simulink model "motor_position_pid_controller"  (R2020a)
settings: Solver=VariableStepAuto  StartTime=0.0  StopTime=10.0  RelTol=1e-3
undefined symbols (not defined in the file or in its folder): B, J, K, L, R
settings Model: DataDictionary=data_dict_motorposition.sldd  Creator=kiran  LastModifiedBy=kiran
settings DataIOCC: SaveOutput=off  SaveTime=off

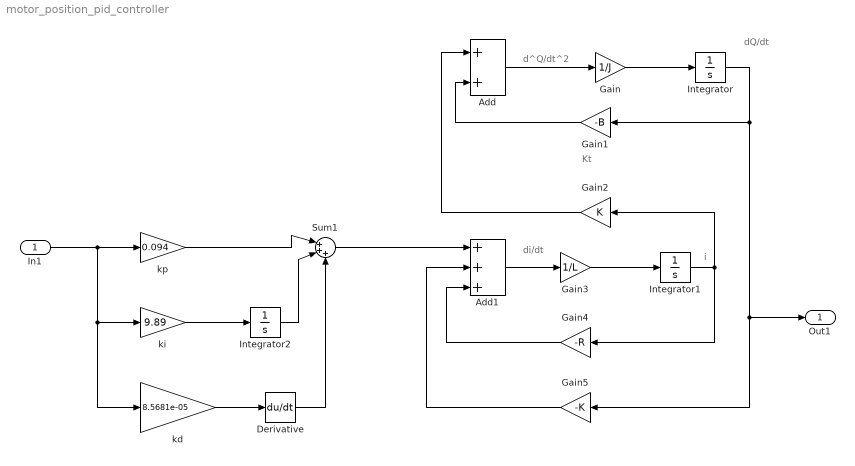
== system motor_position_pid_controller ==
  note: i
  note: dQ/dt
  note: d^Q/dt^2
  note: Kt
  note: di/dt
  In1 : Inport  OutDataTypeStr=double  PortDimensions=1  SampleTime=0
  Add : Sum
  Add1 : Sum  Inputs=+++
  Derivative : Derivative
  Gain : Gain  Gain=1/J
  Gain1 : Gain  Gain=-B
  Gain2 : Gain  Gain=K
  Gain3 : Gain  Gain=1/L
  Gain4 : Gain  Gain=-R
  Gain5 : Gain  Gain=-K
  Integrator : Integrator
  Integrator1 : Integrator
  Integrator2 : Integrator
  Sum1 : Sum  Inputs=|+++
  kd : Gain  Gain=8.5681e-05
  ki : Gain  Gain=9.89
  kp : Gain  Gain=0.094
  Out1 : Outport  OutDataTypeStr=double  PortDimensions=1  SampleTime=0
  wires:
  kp/1 -> Sum1/1
  Gain5/1 -> Add1/2
  Add/1 -> Gain/1
  Gain1/1 -> Add/2
  Gain/1 -> Integrator/1
  In1/1 -> kp/1, ki/1, kd/1
  Gain2/1 -> Add/1
  Gain3/1 -> Integrator1/1
  Integrator1/1 -> Gain2/1, Gain4/1
  ki/1 -> Integrator2/1
  Add1/1 -> Gain3/1
  Integrator2/1 -> Sum1/2
  Derivative/1 -> Sum1/3
  Integrator/1 -> Gain1/1, Gain5/1, Out1/1
  Gain4/1 -> Add1/3
  kd/1 -> Derivative/1
  Sum1/1 -> Add1/1
